simulink library "microgridLibrary"  (R2019b)
settings: Solver=VariableStepAuto  StartTime=0.0  StopTime=10.0  RelTol=1e-3
undefined symbols (not defined in the file or in its folder): Aa, BR, D1, Delta, DiscIntNeverNeededParam, Fn, gcbh, Ion, kv, Lithium, Ls, Pa, Pb, Pc, Rs, sps_rtmsupport, StationData, Ts, Ts_Control, Vn, Vnom
libraries: powerlib x80, simulink x29, powerlib_meascontrol x28, sps_avr x5, spsDieselMotorModel x3, electricdrivelib x2, re_lib x1
(part 4 of 6)

== system microgridLibrary/Solar Array (EMT Model)/Inverter Control ==
  On : Inport  PortDimensions=1
  Vabc_prim : Inport  Port=2  PortDimensions=3
  Iabc_prim : Inport  Port=3  PortDimensions=3
  V_PV : Inport  Port=4  PortDimensions=1
  I_PV : Inport  Port=5  PortDimensions=1
  Vdc_meas : Inport  Port=6  PortDimensions=1
  Current Regulator : Subsystem
  Iq_ref : Constant  Value=0
  MPPT Parameters : Subsystem
  "MPPT Controller using Perturbe & Observe technique " : MATLAB Function  TreatAsAtomicUnit=on
  Mux : Mux  Inputs=2
  Overmodulation : powerlib_meascontrol/Pulse & Signal Generators/Overmodulation  OverModType=Flat top
      settings: SourceProductName=Simscape Electrical  SourceProductBaseCode=PS
  PLL & Measurements : Subsystem
  Switch : Switch  Criteria=u2 ~= 0
  Uabc_ref Generation max (m) = 1 : Subsystem
  Unit Delay : UnitDelay  SampleTime=Ts_Control  HasFrameUpgradeWarning=on
  VDC Regulator : Subsystem
  Vnom_dc1 : Constant  Value=Vnom_dc
  Uref : Outport  VectorParamsAs1DForOutWhenUnconnected=off
  wires:
  PLL & Measurements/1(wt) -> Uabc_ref Generation max (m) = 1/1(wt)
  Current Regulator/1(VdVq_conv) -> Uabc_ref Generation max (m) = 1/2(VdVq_conv)
  Iq_ref/1 -> Mux/2
  Mux/1 -> Current Regulator/3(IdIq_ref)
  PLL & Measurements/3(IdIq_prim) -> Current Regulator/2(IdIq_meas)
  PLL & Measurements/2(VdVq_prim) -> Current Regulator/1(VdVq_meas)
  Vabc_prim/1 -> PLL & Measurements/1(Vabc_prim)
  Iabc_prim/1 -> PLL & Measurements/2(Iabc_prim)
  Overmodulation/1 -> Uref/1
  Vdc_meas/1 -> VDC Regulator/1(Vdc_meas)
  VDC Regulator/1(Id_ref) -> Mux/1
  V_PV/1 -> "MPPT Controller using Perturbe & Observe technique "/3(V)
  I_PV/1 -> "MPPT Controller using Perturbe & Observe technique "/4(I)
  MPPT Parameters/1(Param) -> "MPPT Controller using Perturbe & Observe technique "/1(Param)
  On/1 -> "MPPT Controller using Perturbe & Observe technique "/2(Enabled), Switch/2
  Unit Delay/1 -> Overmodulation/1
  "MPPT Controller using Perturbe & Observe technique "/1(D) -> Switch/1
  Switch/1 -> VDC Regulator/2(Vdc_ref)
  Vnom_dc1/1 -> Switch/3
  Uabc_ref Generation max (m) = 1/1(Uabc_ref) -> Unit Delay/1

== system microgridLibrary/Solar Array (EMT Model)/Measures ==
  Grid : Inport
  PV : Inport  Port=2
  Bus Creator : BusCreator  Inputs=2
  Bus Creator1 : BusCreator  Inputs=4
  Bus Selector2 : BusSelector  OutputSignals=Vabc,Iabc
  "Power (3ph, Instantaneous)" : powerlib_meascontrol/Measurements/Power (3ph, Instantaneous)
      settings: SourceProductName=Simscape Electrical
  m : Outport  VectorParamsAs1DForOutWhenUnconnected=off
  wires:
  Bus Selector2/1 -> "Power (3ph, Instantaneous)"/1, Bus Creator1/1  "<Vabc>"
  Bus Selector2/2 -> "Power (3ph, Instantaneous)"/2, Bus Creator1/2  "<Iabc>"
  "Power (3ph, Instantaneous)"/1 -> Bus Creator1/3  "P"
  Bus Creator/1 -> m/1
  PV/1 -> Bus Creator/2  "PV"
  Grid/1 -> Bus Selector2/1
  "Power (3ph, Instantaneous)"/2 -> Bus Creator1/4  "Q"
  Bus Creator1/1 -> Bus Creator/1  "Grid"

== system microgridLibrary/Variable Load/Dynamic Load Control ==
  P0 : Inport
  Fcn : Fcn  Expr=sqrt(1/u(1)-1)
  Mux : Mux  Inputs=2
  Product : Product
  Summer1 : Constant  Value=PF
  PQ : Outport  VectorParamsAs1DForOutWhenUnconnected=off
  wires:
  Summer1/1 -> Fcn/1
  Fcn/1 -> Product/2
  P0/1 -> Product/1, Mux/1
  Mux/1 -> PQ/1
  Product/1 -> Mux/2  "Qo"

== system microgridLibrary/Diesel Generator (Full Genset Controls)/Continuous/Automatic Generator Controls ==
  Mode : Inport
  PQwv_ref : Inport  Port=2
  GenM : Inport  Port=3
  Demux : Demux  Outputs=2
  "Direct wref, Vref" : Selector  InputPortWidth=4  IndexOptions=Index vector (dialog)  Indices=[3 4]  OutputSizes=1
  Multiport Switch : MultiPortSwitch  DataPortOrder=Zero-based contiguous  zeroidx=on
  PQ Control : Subsystem
  PV Control : Subsystem
  wref : Outport  VectorParamsAs1DForOutWhenUnconnected=off
  vref : Outport  Port=2  VectorParamsAs1DForOutWhenUnconnected=off
  wires:
  Mode/1 -> Multiport Switch/1
  PQwv_ref/1 -> PV Control/1(PQ_wv_ref), "Direct wref, Vref"/1, PQ Control/1(PQ_wv_ref)
  GenM/1 -> PV Control/2(GenM), PQ Control/2(GenM)
  "Direct wref, Vref"/1 -> Multiport Switch/2
  PQ Control/1("wref, Vref") -> Multiport Switch/3
  PV Control/1("wref, Vref") -> Multiport Switch/4
  Multiport Switch/1 -> Demux/1
  Demux/1 -> wref/1
  Demux/2 -> vref/1

== system microgridLibrary/Diesel Generator (Full Genset Controls)/Continuous/Generator Measures ==
  m : Inport
  Bus Selector : BusSelector  OutputSignals="dq0 components.Stator voltage  vq (pu),dq0 components.Stator voltage  vd (pu)"  OutputAsBus=on
  Bus Selector1 : BusSelector  OutputSignals="Mechanical.Rotor speed  wm  (pu),dq0 components.Field current  ifd (pu)"
  Fcn1 : Fcn  Expr=sqrt(u(1)^2 + u(2)^2)
  Ifd : Outport  VectorParamsAs1DForOutWhenUnconnected=off
  Vt : Outport  Port=2  VectorParamsAs1DForOutWhenUnconnected=off
  wm : Outport  Port=3  VectorParamsAs1DForOutWhenUnconnected=off
  wires:
  Fcn1/1 -> Vt/1
  Bus Selector1/2 -> Ifd/1  "<Field current  ifd (pu)>"
  Bus Selector/1 -> Fcn1/1
  m/1 -> Bus Selector/1, Bus Selector1/1
  Bus Selector1/1 -> wm/1  "<Rotor speed  wm  (pu)>"

== system microgridLibrary/Diesel Generator (Full Genset Controls)/Continuous/Selected Measurements ==
  m : Inport
  Bus Creator : BusCreator  Inputs=7
  Bus Selector : BusSelector  OutputSignals="Mechanical.Electrical power  Pe (pu),Mechanical.Rotor speed  wm  (pu),Output active power   Peo (pu),Output reactive power  Qeo (pu)"
  to W : Gain  Gain=Pn
  to W1 : Gain  Gain=Pn
  to W2 : Gain  Gain=Pn
  sm : Outport  VectorParamsAs1DForOutWhenUnconnected=off
  wires:
  m/1 -> Bus Selector/1
  Bus Selector/4 -> to W2/1, Bus Creator/5  "<Output reactive power  Qeo (pu)>"
  Bus Selector/1 -> Bus Creator/2, to W/1  "<Electrical power  Pe (pu)>"
  Bus Selector/3 -> to W1/1, Bus Creator/4  "<Output active power   Peo (pu)>"
  to W/1 -> Bus Creator/1  "Electrical Power (W)"
  Bus Creator/1 -> sm/1
  Bus Selector/2 -> Bus Creator/3  "<Rotor speed  wm  (pu)>"
  to W1/1 -> Bus Creator/6  "Active Power (W)"
  to W2/1 -> Bus Creator/7  "Reactive Power (W)"

== system microgridLibrary/Diesel Generator (Full Genset Controls)/Discrete/Automatic Generator Controls ==
  Mode : Inport
  PQwv_ref : Inport  Port=2  SampleTime=Ts
  GenM : Inport  Port=3
  Demux : Demux  Outputs=2
  "Direct wref, Vref" : Selector  InputPortWidth=4  IndexOptions=Index vector (dialog)  Indices=[3 4]  OutputSizes=1
  Multiport Switch : MultiPortSwitch  DataPortOrder=Zero-based contiguous  zeroidx=on
  PQ Control : Subsystem
  PV Control : Subsystem
  wref : Outport  VectorParamsAs1DForOutWhenUnconnected=off
  vref : Outport  Port=2  VectorParamsAs1DForOutWhenUnconnected=off
  wires:
  Mode/1 -> Multiport Switch/1
  PQwv_ref/1 -> PV Control/1(PQ_wv_ref), "Direct wref, Vref"/1, PQ Control/1(PQ_wv_ref)
  GenM/1 -> PV Control/2(GenM), PQ Control/2(GenM)
  "Direct wref, Vref"/1 -> Multiport Switch/2
  PQ Control/1("wref, Vref") -> Multiport Switch/3
  PV Control/1("wref, Vref") -> Multiport Switch/4
  Multiport Switch/1 -> Demux/1
  Demux/1 -> wref/1
  Demux/2 -> vref/1

== system microgridLibrary/Diesel Generator (Full Genset Controls)/Discrete/Diesel Engine Governor ==
  note: ACTUATOR
  wref (pu) : Inport  SampleTime=Ts
  w (pu) : Inport  Port=2  SampleTime=Ts
  CONTROL SYSTEM : Subsystem
      mask Display: fprintf('(Tr3s + 1)\n-------------------------\n(1+sTr1 + s^2 Tr1*Tr2)');
  ENGINE Td : Delay  DelayLength=ceil(Td/Ts)  InitialCondition=Pm0
  Gain K : Gain  Gain=K  SaturateOnIntegerOverflow=on  OutDataTypeStr=Inherit: Same as input  ParamDataTypeStr=Inherit: Same as input
  Integrator : DiscreteIntegrator  InitialCondition=Pm0  SampleTime=Ts  LimitOutput=on  UpperSaturationLimit=Tlim(2)  LowerSaturationLimit=Tlim(1)  ICPrevOutput=DiscIntNeverNeededParam  ICPrevScaledInput=DiscIntNeverNeededParam
  Product : Product  SaturateOnIntegerOverflow=on  InputSameDT=on  OutDataTypeStr=Inherit: Same as first input
  Sum : Sum  Inputs=+-  SaturateOnIntegerOverflow=on  InputSameDT=on  OutDataTypeStr=Inherit: Same as first input
  TF1 : Subsystem
      mask Display: fprintf('(1 + s Ta1)\n------------\n(1 + s Ta2)');
  TF2 : Subsystem
      mask Display: fprintf('1\n------------\n(1 + s Ta3)');
  Pmec (pu) : Outport  InitialOutput=0  VectorParamsAs1DForOutWhenUnconnected=off
  wires:
  Gain K/1 -> TF1/1(In1)
  Sum/1 -> CONTROL SYSTEM/1(In1)
  CONTROL SYSTEM/1(Out1) -> Gain K/1
  TF1/1(Out1) -> TF2/1(In1)
  w (pu)/1 -> Product/2, Sum/2
  ENGINE Td/1 -> Product/1
  wref (pu)/1 -> Sum/1
  Product/1 -> Pmec (pu)/1
  TF2/1(Out1) -> Integrator/1
  Integrator/1 -> ENGINE Td/1  "Torque"

== system microgridLibrary/Diesel Generator (Full Genset Controls)/Discrete/Generator Measures ==
  m : Inport
  Bus Selector : BusSelector  OutputSignals="dq0 components.Stator voltage  vq (pu),dq0 components.Stator voltage  vd (pu)"  OutputAsBus=on
  Bus Selector1 : BusSelector  OutputSignals="Mechanical.Rotor speed  wm  (pu),dq0 components.Field current  ifd (pu)"
  Fcn1 : Fcn  Expr=sqrt(u(1)^2 + u(2)^2)
  Ifd : Outport  VectorParamsAs1DForOutWhenUnconnected=off
  Vt : Outport  Port=2  VectorParamsAs1DForOutWhenUnconnected=off
  wm : Outport  Port=3  VectorParamsAs1DForOutWhenUnconnected=off
  wires:
  Bus Selector1/1 -> wm/1  "<Rotor speed  wm  (pu)>"
  m/1 -> Bus Selector1/1, Bus Selector/1
  Fcn1/1 -> Vt/1
  Bus Selector/1 -> Fcn1/1
  Bus Selector1/2 -> Ifd/1  "<Field current  ifd (pu)>"

== system microgridLibrary/Diesel Generator (Full Genset Controls)/Discrete/Selected Measurements ==
  m : Inport
  Bus Creator : BusCreator  Inputs=7
  Bus Selector : BusSelector  OutputSignals="Mechanical.Electrical power  Pe (pu),Mechanical.Rotor speed  wm  (pu),Output active power   Peo (pu),Output reactive power  Qeo (pu)"
  to W : Gain  Gain=Pn
  to W1 : Gain  Gain=Pn
  to W2 : Gain  Gain=Pn
  sm : Outport  VectorParamsAs1DForOutWhenUnconnected=off
  wires:
  to W2/1 -> Bus Creator/7  "Reactive Power (W)"
  to W1/1 -> Bus Creator/6  "Active Power (W)"
  Bus Selector/2 -> Bus Creator/3  "<Rotor speed  wm  (pu)>"
  Bus Creator/1 -> sm/1
  to W/1 -> Bus Creator/1  "Electrical Power (W)"
  Bus Selector/3 -> Bus Creator/4, to W1/1  "<Output active power   Peo (pu)>"
  Bus Selector/1 -> to W/1, Bus Creator/2  "<Electrical power  Pe (pu)>"
  Bus Selector/4 -> Bus Creator/5, to W2/1  "<Output reactive power  Qeo (pu)>"
  m/1 -> Bus Selector/1

== system microgridLibrary/Diesel Generator (Simple Controls)/Continuous/Generator Measures ==
  m : Inport
  Bus Selector : BusSelector  OutputSignals="dq0 components.Stator voltage  vq (pu),dq0 components.Stator voltage  vd (pu)"  OutputAsBus=on
  Bus Selector1 : BusSelector  OutputSignals="Mechanical.Rotor speed  wm  (pu),dq0 components.Field current  ifd (pu)"
  Fcn1 : Fcn  Expr=sqrt(u(1)^2 + u(2)^2)
  Ifd : Outport  VectorParamsAs1DForOutWhenUnconnected=off
  Vt : Outport  Port=2  VectorParamsAs1DForOutWhenUnconnected=off
  wm : Outport  Port=3  VectorParamsAs1DForOutWhenUnconnected=off
  wires:
  Bus Selector1/1 -> wm/1  "<Rotor speed  wm  (pu)>"
  m/1 -> Bus Selector1/1, Bus Selector/1
  Bus Selector/1 -> Fcn1/1
  Bus Selector1/2 -> Ifd/1  "<Field current  ifd (pu)>"
  Fcn1/1 -> Vt/1

== system microgridLibrary/Diesel Generator (Simple Controls)/Continuous/Selected Measurements ==
  m : Inport
  Bus Creator : BusCreator  Inputs=7
  Bus Selector : BusSelector  OutputSignals="Mechanical.Electrical power  Pe (pu),Mechanical.Rotor speed  wm  (pu),Output active power   Peo (pu),Output reactive power  Qeo (pu)"
  to W : Gain  Gain=Pn
  to W1 : Gain  Gain=Pn
  to W2 : Gain  Gain=Pn
  sm : Outport  VectorParamsAs1DForOutWhenUnconnected=off
  wires:
  to W2/1 -> Bus Creator/7  "Reactive Power (W)"
  to W1/1 -> Bus Creator/6  "Active Power (W)"
  Bus Selector/2 -> Bus Creator/3  "<Rotor speed  wm  (pu)>"
  Bus Creator/1 -> sm/1
  to W/1 -> Bus Creator/1  "Electrical Power (W)"
  Bus Selector/3 -> Bus Creator/4, to W1/1  "<Output active power   Peo (pu)>"
  Bus Selector/1 -> to W/1, Bus Creator/2  "<Electrical power  Pe (pu)>"
  Bus Selector/4 -> Bus Creator/5, to W2/1  "<Output reactive power  Qeo (pu)>"
  m/1 -> Bus Selector/1

== system microgridLibrary/Diesel Generator (Simple Controls)/Discrete/Diesel Engine Governor ==
  note: ACTUATOR
  wref (pu) : Inport  SampleTime=Ts
  w (pu) : Inport  Port=2  SampleTime=Ts
  CONTROL SYSTEM : Subsystem
      mask Display: fprintf('(Tr3s + 1)\n-------------------------\n(1+sTr1 + s^2 Tr1*Tr2)');
  ENGINE Td : Delay  DelayLength=ceil(Td/Ts)  InitialCondition=Pm0
  Gain K : Gain  Gain=K  SaturateOnIntegerOverflow=on  OutDataTypeStr=Inherit: Same as input  ParamDataTypeStr=Inherit: Same as input
  Integrator : DiscreteIntegrator  InitialCondition=Pm0  SampleTime=Ts  LimitOutput=on  UpperSaturationLimit=Tlim(2)  LowerSaturationLimit=Tlim(1)  ICPrevOutput=DiscIntNeverNeededParam  ICPrevScaledInput=DiscIntNeverNeededParam
  Product : Product  SaturateOnIntegerOverflow=on  InputSameDT=on  OutDataTypeStr=Inherit: Same as first input
  Sum : Sum  Inputs=+-  SaturateOnIntegerOverflow=on  InputSameDT=on  OutDataTypeStr=Inherit: Same as first input
  TF1 : Subsystem
      mask Display: fprintf('(1 + s Ta1)\n------------\n(1 + s Ta2)');
  TF2 : Subsystem
      mask Display: fprintf('1\n------------\n(1 + s Ta3)');
  Pmec (pu) : Outport  InitialOutput=0  VectorParamsAs1DForOutWhenUnconnected=off
  wires:
  Integrator/1 -> ENGINE Td/1  "Torque"
  TF2/1(Out1) -> Integrator/1
  Product/1 -> Pmec (pu)/1
  wref (pu)/1 -> Sum/1
  ENGINE Td/1 -> Product/1
  w (pu)/1 -> Sum/2, Product/2
  TF1/1(Out1) -> TF2/1(In1)
  CONTROL SYSTEM/1(Out1) -> Gain K/1
  Sum/1 -> CONTROL SYSTEM/1(In1)
  Gain K/1 -> TF1/1(In1)

== system microgridLibrary/Diesel Generator (Simple Controls)/Discrete/Generator Measures ==
  m : Inport
  Bus Selector : BusSelector  OutputSignals="dq0 components.Stator voltage  vq (pu),dq0 components.Stator voltage  vd (pu)"  OutputAsBus=on
  Bus Selector1 : BusSelector  OutputSignals="Mechanical.Rotor speed  wm  (pu),dq0 components.Field current  ifd (pu)"
  Fcn1 : Fcn  Expr=sqrt(u(1)^2 + u(2)^2)
  Ifd : Outport  VectorParamsAs1DForOutWhenUnconnected=off
  Vt : Outport  Port=2  VectorParamsAs1DForOutWhenUnconnected=off
  wm : Outport  Port=3  VectorParamsAs1DForOutWhenUnconnected=off
  wires:
  Bus Selector1/2 -> Ifd/1  "<Field current  ifd (pu)>"
  Bus Selector/1 -> Fcn1/1
  Fcn1/1 -> Vt/1
  m/1 -> Bus Selector/1, Bus Selector1/1
  Bus Selector1/1 -> wm/1  "<Rotor speed  wm  (pu)>"

== system microgridLibrary/Diesel Generator (Simple Controls)/Discrete/Selected Measurements ==
  m : Inport
  Bus Creator : BusCreator  Inputs=7
  Bus Selector : BusSelector  OutputSignals="Mechanical.Electrical power  Pe (pu),Mechanical.Rotor speed  wm  (pu),Output active power   Peo (pu),Output reactive power  Qeo (pu)"
  to W : Gain  Gain=Pn
  to W1 : Gain  Gain=Pn
  to W2 : Gain  Gain=Pn
  sm : Outport  VectorParamsAs1DForOutWhenUnconnected=off
  wires:
  m/1 -> Bus Selector/1
  Bus Selector/4 -> to W2/1, Bus Creator/5  "<Output reactive power  Qeo (pu)>"
  Bus Selector/1 -> Bus Creator/2, to W/1  "<Electrical power  Pe (pu)>"
  Bus Selector/3 -> to W1/1, Bus Creator/4  "<Output active power   Peo (pu)>"
  to W/1 -> Bus Creator/1  "Electrical Power (W)"
  Bus Creator/1 -> sm/1
  Bus Selector/2 -> Bus Creator/3  "<Rotor speed  wm  (pu)>"
  to W1/1 -> Bus Creator/6  "Active Power (W)"
  to W2/1 -> Bus Creator/7  "Reactive Power (W)"

== system microgridLibrary/Energy Storage (PQ Model)/Charge Limits/Overcharge Check ==
  SOC (%) : Inport
  Pin : Inport  Port=2
  Qin : Inport  Port=3
  Backlash : Backlash  BacklashWidth=1e-3  InitialOutput=Initial_kWh_pc  ZeroCross=off
  Compare To Constant : simulink/Logic and Bit Operations/Compare To Constant  relop=>  const=UpChrgLim  OutDataTypeStr=boolean
  Compare To Zero : simulink/Logic and Bit Operations/Compare To Zero  relop=<=  OutDataTypeStr=boolean
  Constant : Constant  Value=0
  Constant1 : Constant  Value=0
  Logical Operator : Logic  AllPortsSameDT=off  OutDataTypeStr=boolean
  Switch : Switch  Criteria=u2 ~= 0
  Switch1 : Switch  Criteria=u2 ~= 0
  Pout : Outport  VectorParamsAs1DForOutWhenUnconnected=off
  Qout : Outport  Port=2  VectorParamsAs1DForOutWhenUnconnected=off
  wires:
  Backlash/1 -> Compare To Constant/1
  Switch1/1 -> Qout/1
  Constant1/1 -> Switch1/1
  Qin/1 -> Switch1/3
  Compare To Zero/1 -> Logical Operator/2
  Switch/1 -> Pout/1
  Pin/1 -> Switch/3, Compare To Zero/1
  SOC (%)/1 -> Backlash/1
  Constant/1 -> Switch/1
  Logical Operator/1 -> Switch/2, Switch1/2
  Compare To Constant/1 -> Logical Operator/1

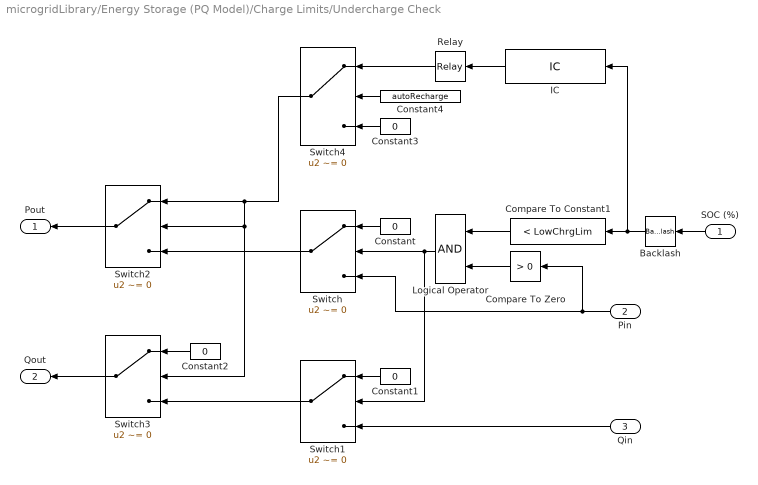
== system microgridLibrary/Energy Storage (PQ Model)/Charge Limits/Undercharge Check ==
  SOC (%) : Inport
  Pin : Inport  Port=2
  Qin : Inport  Port=3
  Backlash : Backlash  BacklashWidth=1e-3  InitialOutput=Initial_kWh_pc  ZeroCross=off
  Compare To Constant1 : simulink/Logic and Bit Operations/Compare To Constant  relop=<  const=LowChrgLim  OutDataTypeStr=boolean
  Compare To Zero : simulink/Logic and Bit Operations/Compare To Zero  relop=>  OutDataTypeStr=boolean
  Constant{,1..3} (4 alike) : Constant  Value=0
  Constant4 : Constant  Value=autoRecharge
  IC : InitialCondition  Value=RechargeSOC
  Logical Operator : Logic  AllPortsSameDT=off  OutDataTypeStr=boolean
  Relay : Relay  OnSwitchValue=RechargeSOC  OffSwitchValue=LowChrgLim  OnOutputValue=0  OffOutputValue=-Precharge/100*Pnom
  Switch{,1..4} (5 alike) : Switch  Criteria=u2 ~= 0
  Pout : Outport  VectorParamsAs1DForOutWhenUnconnected=off
  Qout : Outport  Port=2  VectorParamsAs1DForOutWhenUnconnected=off
  wires:
  Constant4/1 -> Switch4/2
  Constant3/1 -> Switch4/3
  Relay/1 -> Switch4/1
  Constant2/1 -> Switch3/1
  Switch1/1 -> Switch3/3
  Switch3/1 -> Qout/1
  Switch2/1 -> Pout/1
  Switch/1 -> Switch2/3
  IC/1 -> Relay/1
  Switch4/1 -> Switch3/2, Switch2/2, Switch2/1
  Backlash/1 -> Compare To Constant1/1, IC/1
  Qin/1 -> Switch1/3
  Constant1/1 -> Switch1/1
  Compare To Constant1/1 -> Logical Operator/1
  Logical Operator/1 -> Switch1/2, Switch/2
  Constant/1 -> Switch/1
  SOC (%)/1 -> Backlash/1
  Pin/1 -> Compare To Zero/1, Switch/3
  Compare To Zero/1 -> Logical Operator/2

== system microgridLibrary/Energy Storage (PQ Model)/Power Measures/EMT ==
  "Power (3ph, Instantaneous)" : powerlib_meascontrol/Measurements/Power (3ph, Instantaneous)
      settings: SourceProductName=Simscape Electrical
  Three-Phase V-I Measurement : powerlib/Measurements/Three-Phase V-I Measurement  VoltageMeasurement=phase-to-ground  SetLabelV=off  LabelV=Vabc  Vpu=off  VpuLL=off  CurrentMeasurement=yes  SetLabelI=off  LabelI=Iabc  Ipu=off  Pbase=100e6  Vbase=500e3  OutputType=Complex  PhasorSimulation=on  PSBequivalent=0
      settings: SourceProductName=Simscape Electrical
  A : PMIOPort  Side=Left
  a : PMIOPort  Port=2  Side=Right
  B : PMIOPort  Port=3  Side=Left
  b : PMIOPort  Port=4  Side=Right
  C : PMIOPort  Port=5  Side=Left
  c : PMIOPort  Port=6  Side=Right
  P : Outport  VectorParamsAs1DForOutWhenUnconnected=off
  Q : Outport  Port=2  VectorParamsAs1DForOutWhenUnconnected=off
  wires:
  Three-Phase V-I Measurement/2 -> "Power (3ph, Instantaneous)"/2
  Three-Phase V-I Measurement/1 -> "Power (3ph, Instantaneous)"/1
  "Power (3ph, Instantaneous)"/1 -> P/1
  "Power (3ph, Instantaneous)"/2 -> Q/1
  connections:
  Three-Phase V-I Measurement/RConn1 -- a/RConn1
  b/RConn1 -- Three-Phase V-I Measurement/RConn2
  A/RConn1 -- Three-Phase V-I Measurement/LConn1
  Three-Phase V-I Measurement/LConn2 -- B/RConn1
  c/RConn1 -- Three-Phase V-I Measurement/RConn3
  C/RConn1 -- Three-Phase V-I Measurement/LConn3

== system microgridLibrary/Energy Storage (PQ Model)/Power Measures/Phasor ==
  "Power (3ph, Phasor)" : powerlib_meascontrol/Measurements/Power (3ph, Phasor)
      settings: SourceProductName=Simscape Electrical  SourceProductBaseCode=PS
  Three-Phase V-I Measurement : powerlib/Measurements/Three-Phase V-I Measurement  VoltageMeasurement=phase-to-ground  SetLabelV=off  LabelV=Vabc  Vpu=off  VpuLL=off  CurrentMeasurement=yes  SetLabelI=off  LabelI=Iabc  Ipu=off  Pbase=100e6  Vbase=500e3  OutputType=Complex  PhasorSimulation=on  PSBequivalent=0
      settings: SourceProductName=Simscape Electrical
  A : PMIOPort  Side=Left
  a : PMIOPort  Port=2  Side=Right
  B : PMIOPort  Port=3  Side=Left
  b : PMIOPort  Port=4  Side=Right
  C : PMIOPort  Port=5  Side=Left
  c : PMIOPort  Port=6  Side=Right
  P : Outport  VectorParamsAs1DForOutWhenUnconnected=off
  Q : Outport  Port=2  VectorParamsAs1DForOutWhenUnconnected=off
  wires:
  "Power (3ph, Phasor)"/2 -> Q/1
  "Power (3ph, Phasor)"/1 -> P/1
  Three-Phase V-I Measurement/1 -> "Power (3ph, Phasor)"/1
  Three-Phase V-I Measurement/2 -> "Power (3ph, Phasor)"/2
  connections:
  C/RConn1 -- Three-Phase V-I Measurement/LConn3
  c/RConn1 -- Three-Phase V-I Measurement/RConn3
  Three-Phase V-I Measurement/LConn2 -- B/RConn1
  A/RConn1 -- Three-Phase V-I Measurement/LConn1
  b/RConn1 -- Three-Phase V-I Measurement/RConn2
  Three-Phase V-I Measurement/RConn1 -- a/RConn1

== system microgridLibrary/Fault /Fault A/Model ==
  "gate " : Inport
  Uswitch : Inport  Port=2
  C4 : Constant  Value=BR.com
  Data Type Conversion : DataTypeConversion  OutDataTypeStr=double  SaturateOnIntegerOverflow=on  RndMeth=Zero
  Switch3 : Switch  Threshold=0.5  ZeroCross=off  InputSameDT=on
  This signal is not used : Terminator
  Timer : Subsystem  DialogController=POWERSYS.PowerSysDialog  mask(Timer){t=BR.SwitchingTimes, e=BR.switchings}
      mask prompts: t "Time (s):"; e "Amplitude:"
      mask help:
      | Generates a signal changing at specified times.
      |
      | If a signal value is not specified at time zero, the output is kept at 0 until the first specified transition time.
      mask init:
      | tt=t;
      | sv=e;
      | if isempty(tt) | isempty(sv)
      | 	% probably during the load process when under a masked block.
      | 	tt=0;
      | 	sv=1;
      | end
      | %
      | if length(sv) ~= length(tt),
      |    Erreur.message = 'The vectors specifying the time and amplitude pairs must have the same length.';
      |    Erreur.identifier = 'SimscapePowerSystemsST:TimerBlock:ParameterError';
      |    powericon('psberror',Erreur.message,Erreur.identifier,'NoUiwait');
      | end
      | if tt(1)~=0,
      |    tt=[0 tt];
      |    sv=[~sv(1) sv];
      | end
      | n=length(tt);
      | vec_dt=[tt,0]-[0,tt] ;
      | vec_dt=vec_dt(2:n);
      | if any(vec_dt<=0)
      |    Erreur.message = 'All transition times must be in increasing order.';
      |    Erreur.identifier = 'SimscapePowerSystemsST:TimerBlock:ParameterError';
      |    powericon('psberror',Erreur.message,Erreur.identifier,'NoUiwait');
      | end
      | tv=[-1,tt(1),reshape(repmat(reshape(tt(2:end),1,length(tt)-1),2,1),1,2*length(tt)-2),tt(end)+1];
      | %sv=(sv(:)'~=0);
      | opv=[sv(1),reshape(repmat(sv(1:end-1),2,1),1,2*length(sv)-2),sv(end),sv(end)];
      | 
      | power_initmask();
      mask Help: helpview(psbhelp)
      mask Display: plot( tv(2:end-1), opv(2:end-1) )
  gate : Outport  VectorParamsAs1DForOutWhenUnconnected=off
  wires:
  Uswitch/1 -> This signal is not used/1
  C4/1 -> Switch3/2
  Timer/1(Out) -> Switch3/3
  Data Type Conversion/1 -> Switch3/1
  Switch3/1 -> gate/1
  "gate "/1 -> Data Type Conversion/1

== system microgridLibrary/Fault /Fault B/Model ==
  "gate " : Inport
  Uswitch : Inport  Port=2
  C4 : Constant  Value=BR.com
  Data Type Conversion : DataTypeConversion  OutDataTypeStr=double  SaturateOnIntegerOverflow=on  RndMeth=Zero
  Switch3 : Switch  Threshold=0.5  ZeroCross=off  InputSameDT=on
  This signal is not used : Terminator
  Timer : Subsystem  DialogController=POWERSYS.PowerSysDialog  mask(Timer){t=BR.SwitchingTimes, e=BR.switchings}
      mask prompts: t "Time (s):"; e "Amplitude:"
      mask help:
      | Generates a signal changing at specified times.
      |
      | If a signal value is not specified at time zero, the output is kept at 0 until the first specified transition time.
      mask init: same as microgridLibrary/Fault /Fault A/Model/Timer
      mask Help: helpview(psbhelp)
      mask Display: plot( tv(2:end-1), opv(2:end-1) )
  gate : Outport  VectorParamsAs1DForOutWhenUnconnected=off
  wires:
  Uswitch/1 -> This signal is not used/1
  C4/1 -> Switch3/2
  Timer/1(Out) -> Switch3/3
  Data Type Conversion/1 -> Switch3/1
  Switch3/1 -> gate/1
  "gate "/1 -> Data Type Conversion/1

== system microgridLibrary/Fault /Fault C/Model ==
  "gate " : Inport
  Uswitch : Inport  Port=2
  C4 : Constant  Value=BR.com
  Data Type Conversion : DataTypeConversion  OutDataTypeStr=double  SaturateOnIntegerOverflow=on  RndMeth=Zero
  Switch3 : Switch  Threshold=0.5  ZeroCross=off  InputSameDT=on
  This signal is not used : Terminator
  Timer : Subsystem  DialogController=POWERSYS.PowerSysDialog  mask(Timer){t=BR.SwitchingTimes, e=BR.switchings}
      mask prompts: t "Time (s):"; e "Amplitude:"
      mask help:
      | Generates a signal changing at specified times.
      |
      | If a signal value is not specified at time zero, the output is kept at 0 until the first specified transition time.
      mask init: same as microgridLibrary/Fault /Fault A/Model/Timer
      mask Help: helpview(psbhelp)
      mask Display: plot( tv(2:end-1), opv(2:end-1) )
  gate : Outport  VectorParamsAs1DForOutWhenUnconnected=off
  wires:
  Uswitch/1 -> This signal is not used/1
  C4/1 -> Switch3/2
  Timer/1(Out) -> Switch3/3
  Data Type Conversion/1 -> Switch3/1
  Switch3/1 -> gate/1
  "gate "/1 -> Data Type Conversion/1

== system microgridLibrary/Grid Source Phasor Load Flow/Model/Initial Voltage ==
  Constant3 : Constant  Value=0
  Integrator : Integrator  InitialCondition=0.95
  Aa : Outport
  wires:
  Constant3/1 -> Integrator/1
  Integrator/1 -> Aa/1

== system microgridLibrary/Grid-Connected Battery (EMT with Simple Controls)/Battery Controller/Compute PQ ==
  m : Inport
  Bus Selector : BusSelector  OutputSignals=Vabc,Iabc
  Mux : Mux  Inputs=2
  "Power (3ph, Instantaneous)" : powerlib_meascontrol/Measurements/Power (3ph, Instantaneous)
      settings: SourceProductName=Simscape Electrical
  to PU : Gain  Gain=1/Pnom
  "to PU " : Gain  Gain=1/Pnom
  PQm : Outport  VectorParamsAs1DForOutWhenUnconnected=off
  wires:
  Bus Selector/1 -> "Power (3ph, Instantaneous)"/1  "<Vabc>"
  "Power (3ph, Instantaneous)"/2 -> "to PU "/1
  Bus Selector/2 -> "Power (3ph, Instantaneous)"/2  "<Iabc>"
  "Power (3ph, Instantaneous)"/1 -> to PU/1
  m/1 -> Bus Selector/1
  to PU/1 -> Mux/1
  "to PU "/1 -> Mux/2
  Mux/1 -> PQm/1

== system microgridLibrary/Grid-Connected Battery (EMT with Simple Controls)/Battery Controller/P,Q Control  ==
  PQref : Inport
  m : Inport  Port=2
  Active Controller : simulink/Continuous/PID Controller  Controller=PI  Form=Parallel  TimeDomain=Discrete-time  SampleTime=Ts_Control  IntegratorMethod=Forward Euler  FilterMethod=Forward Euler  ControllerParametersSource=internal  P=1  I=10  D=0  UseFilter=on  N=100  TunerSelectOption=Transfer Function Based (PID Tuner App)  InitialConditionSource=internal  InitialConditionForIntegrator=0  InitialConditionForFilter=0  DifferentiatorICPrevScaledInput=0  ExternalReset=none  TrackingMode=off  Kt=1  LimitOutput=on  UpperSaturationLimit=1.5  LowerSaturationLimit=-1.5  LinearizeAsGain=off  AntiWindupMode=clamping  Kb=1  POutMin=[]  POutMax=[]  IOutMin=[]  IOutMax=[]  DOutMin=[]  DOutMax=[]  NOutMin=[]  NOutMax=[]  SumOutMin=[]  SumOutMax=[]  SaturationOutMin=[]  SaturationOutMax=[]  PParamMin=[]  PParamMax=[]  IParamMin=[]  IParamMax=[]  DParamMin=[]  DParamMax=[]  NParamMin=[]  NParamMax=[]  KbParamMin=[]  KbParamMax=[]  KtParamMin=[]  KtParamMax=[]  KbOutMin=[]  KbOutMax=[]  KtOutMin=[]  KtOutMax=[]  IntegratorOutMin=[]  IntegratorOutMax=[]  FilterOutMin=[]  FilterOutMax=[]  SumI1OutMin=[]  SumI1OutMax=[]  SumI2OutMin=[]  SumI2OutMax=[]  SumI3OutMin=[]  SumI3OutMax=[]  SumI4OutMin=[]  SumI4OutMax=[]  SumDOutMin=[]  SumDOutMax=[]  DifferentiatorOutMin=[]  DifferentiatorOutMax=[]  FilterDiffOutCoefMin=[]  FilterDiffOutCoefMax=[]  ReciprocalOutMin=[]  ReciprocalOutMax=[]  SumDenOutMin=[]  SumDenOutMax=[]  SumNumOutMin=[]  SumNumOutMax=[]  DivideOutMin=[]  DivideOutMax=[]  IntegratorContinuousStateAttributes=''  IntegratorStateMustResolveToSignalObject=off  IntegratorRTWStateStorageClass=Auto  FilterContinuousStateAttributes=''  FilterStateMustResolveToSignalObject=off  FilterRTWStateStorageClass=Auto  ParallelPVariant=InternalParameters  IdealPVariant=Disabled  IVariant=InternalParameters  DVariant=Disabled  IntegratorVariant=Discrete  SatVariant=Enabled  AWVariant=DiscClampingParallel  PCopyVariant=Disabled  TRVariant=Disabled  FdbkBlocksVariant=Forward  IdealPFdbkVariant=Disabled  SatFdbkVariant=Disabled  DerivativeFilterVariant=Disabled  NVariant=Disabled  NCopyVariant=Disabled_SignalSpec  FilterICVariant=Disabled  IntegratorICVariant=InternalICs  ExternalResetVariant=Disabled  TRSumVariant=Passthrough  SumFdbkVariant=Disabled  SumVariant=Sum_PI
  Demux : Demux  Outputs=2
  Demux1 : Demux  Outputs=2
  Mux : Mux  Inputs=2
  Reactive Controller : simulink/Continuous/PID Controller  Controller=PI  Form=Parallel  TimeDomain=Discrete-time  SampleTime=Ts_Control  IntegratorMethod=Forward Euler  FilterMethod=Forward Euler  ControllerParametersSource=internal  P=1  I=10  D=0  UseFilter=on  N=100  TunerSelectOption=Transfer Function Based (PID Tuner App)  InitialConditionSource=internal  InitialConditionForIntegrator=0  InitialConditionForFilter=0  DifferentiatorICPrevScaledInput=0  ExternalReset=none  TrackingMode=off  Kt=1  LimitOutput=on  UpperSaturationLimit=1.5  LowerSaturationLimit=-1.5  LinearizeAsGain=off  AntiWindupMode=clamping  Kb=1  POutMin=[]  POutMax=[]  IOutMin=[]  IOutMax=[]  DOutMin=[]  DOutMax=[]  NOutMin=[]  NOutMax=[]  SumOutMin=[]  SumOutMax=[]  SaturationOutMin=[]  SaturationOutMax=[]  PParamMin=[]  PParamMax=[]  IParamMin=[]  IParamMax=[]  DParamMin=[]  DParamMax=[]  NParamMin=[]  NParamMax=[]  KbParamMin=[]  KbParamMax=[]  KtParamMin=[]  KtParamMax=[]  KbOutMin=[]  KbOutMax=[]  KtOutMin=[]  KtOutMax=[]  IntegratorOutMin=[]  IntegratorOutMax=[]  FilterOutMin=[]  FilterOutMax=[]  SumI1OutMin=[]  SumI1OutMax=[]  SumI2OutMin=[]  SumI2OutMax=[]  SumI3OutMin=[]  SumI3OutMax=[]  SumI4OutMin=[]  SumI4OutMax=[]  SumDOutMin=[]  SumDOutMax=[]  DifferentiatorOutMin=[]  DifferentiatorOutMax=[]  FilterDiffOutCoefMin=[]  FilterDiffOutCoefMax=[]  ReciprocalOutMin=[]  ReciprocalOutMax=[]  SumDenOutMin=[]  SumDenOutMax=[]  SumNumOutMin=[]  SumNumOutMax=[]  DivideOutMin=[]  DivideOutMax=[]  IntegratorContinuousStateAttributes=''  IntegratorStateMustResolveToSignalObject=off  IntegratorRTWStateStorageClass=Auto  FilterContinuousStateAttributes=''  FilterStateMustResolveToSignalObject=off  FilterRTWStateStorageClass=Auto  ParallelPVariant=InternalParameters  IdealPVariant=Disabled  IVariant=InternalParameters  DVariant=Disabled  IntegratorVariant=Discrete  SatVariant=Enabled  AWVariant=DiscClampingParallel  PCopyVariant=Disabled  TRVariant=Disabled  FdbkBlocksVariant=Forward  IdealPFdbkVariant=Disabled  SatFdbkVariant=Disabled  DerivativeFilterVariant=Disabled  NVariant=Disabled  NCopyVariant=Disabled_SignalSpec  FilterICVariant=Disabled  IntegratorICVariant=InternalICs  ExternalResetVariant=Disabled  TRSumVariant=Passthrough  SumFdbkVariant=Disabled  SumVariant=Sum_PI
  Sum : Sum  Inputs=|+-
  Sum1 : Sum  Inputs=|-+
  Idq_ref : Outport  VectorParamsAs1DForOutWhenUnconnected=off
  wires:
  Sum1/1 -> Reactive Controller/1
  Sum/1 -> Active Controller/1
  Mux/1 -> Idq_ref/1
  Active Controller/1 -> Mux/1
  Reactive Controller/1 -> Mux/2
  Demux/2 -> Sum1/1  "Qref"
  Demux/1 -> Sum/1  "Pref"
  PQref/1 -> Demux/1
  m/1 -> Demux1/1
  Demux1/1 -> Sum/2
  Demux1/2 -> Sum1/2

== system microgridLibrary/Grid-Connected Battery (EMT with Simple Controls)/Inverter Control/Current Control ==
  wt : Inport
  VdVq_meas : Inport  Port=2  PortDimensions=2
  IdIq_meas : Inport  Port=3  PortDimensions=2
  IdIq_ref : Inport  Port=4  PortDimensions=2
  Current Regulator : Subsystem
  Uabc_ref Generation max (m) = 1 : Subsystem
  Uabc : Outport  VectorParamsAs1DForOutWhenUnconnected=off
  wires:
  Uabc_ref Generation max (m) = 1/1(Uabc_ref) -> Uabc/1
  IdIq_ref/1 -> Current Regulator/3(IdIq_ref)
  IdIq_meas/1 -> Current Regulator/2(IdIq_meas)
  VdVq_meas/1 -> Current Regulator/1(VdVq_meas)
  Current Regulator/1(VdVq_conv) -> Uabc_ref Generation max (m) = 1/2(VdVq_conv)
  wt/1 -> Uabc_ref Generation max (m) = 1/1(wt)

== system microgridLibrary/Grid-Connected Battery (EMT with Simple Controls)/Inverter Control/PLL & Measurements ==
  note: PLL & Measurements
      | ===================
  Vabc_prim : Inport
  Iabc_prim : Inport  Port=2
  PLL (3ph) : powerlib_meascontrol/PLL/PLL (3ph)  Fmin=45  Par_Init="[-0.57  Fnom]"  ParK=[180, 3200, 1]  TcD=Ts_Control  MaxRateChangeFreq=12  FilterCutOffFreq=25  Ts=Ts_Control  AGC=on
      settings: SourceProductName=Simscape Electrical
  Selector1 : Selector  InputPortWidth=3  IndexOptions=Index vector (dialog)  Indices=[1 2]  OutputSizes=1
  Selector2 : Selector  InputPortWidth=3  IndexOptions=Index vector (dialog)  Indices=[1 2]  OutputSizes=1
  Terminator : Terminator
  V->pu : Gain  Gain=1/(Vnom_prim*sqrt(2)/sqrt(3))  SaturateOnIntegerOverflow=on  OutDataTypeStr=Inherit: Same as input  ParamDataTypeStr=Inherit: Same as input
  V->pu1 : Gain  Gain=Vnom_prim*sqrt(3)/Pnom/sqrt(2)  SaturateOnIntegerOverflow=on  OutDataTypeStr=Inherit: Same as input  ParamDataTypeStr=Inherit: Same as input
  abc to dq0 : powerlib_meascontrol/Transformations/abc to dq0  Alignment=90 degrees behind phase A axis
      settings: SourceProductName=Simscape Electrical
  abc to dq1 : powerlib_meascontrol/Transformations/abc to dq0  Alignment=90 degrees behind phase A axis
      settings: SourceProductName=Simscape Electrical
  wt : Outport  VectorParamsAs1DForOutWhenUnconnected=off
  VdVq_prim : Outport  Port=2  VectorParamsAs1DForOutWhenUnconnected=off
  IdIq_prim : Outport  Port=3  VectorParamsAs1DForOutWhenUnconnected=off
  wires:
  V->pu1/1 -> abc to dq1/1
  V->pu/1 -> PLL (3ph)/1, abc to dq0/1
  abc to dq1/1 -> Selector1/1
  Vabc_prim/1 -> V->pu/1
  Iabc_prim/1 -> V->pu1/1
  abc to dq0/1 -> Selector2/1
  Selector2/1 -> VdVq_prim/1
  Selector1/1 -> IdIq_prim/1
  PLL (3ph)/2 -> wt/1, abc to dq1/2, abc to dq0/2
  PLL (3ph)/1 -> Terminator/1

== system microgridLibrary/Grid-Connected Battery (Multi-mode EMT Model)/Battery Controller/Compute PQ ==
  m : Inport
  Bus Selector : BusSelector  OutputSignals=Vabc,Iabc
  Mux : Mux  Inputs=2
  "Power (3ph, Instantaneous)" : powerlib_meascontrol/Measurements/Power (3ph, Instantaneous)
      settings: SourceProductName=Simscape Electrical
  to PU : Gain  Gain=1/Pnom
  "to PU " : Gain  Gain=1/Pnom
  PQm : Outport  VectorParamsAs1DForOutWhenUnconnected=off
  wires:
  Mux/1 -> PQm/1
  "to PU "/1 -> Mux/2
  to PU/1 -> Mux/1
  m/1 -> Bus Selector/1
  "Power (3ph, Instantaneous)"/1 -> to PU/1
  Bus Selector/2 -> "Power (3ph, Instantaneous)"/2  "<Iabc>"
  "Power (3ph, Instantaneous)"/2 -> "to PU "/1
  Bus Selector/1 -> "Power (3ph, Instantaneous)"/1  "<Vabc>"

== system microgridLibrary/Grid-Connected Battery (Multi-mode EMT Model)/Battery Controller/Disable Current Control ==
  Action Port : ActionPort  InitializeStates=reset
  Id_ref : Constant  Value=0
  Iq_ref : Constant  Value=0
  Mux : Mux  Inputs=2
  Idq_ref : Outport  VectorParamsAs1DForOutWhenUnconnected=off
  wires:
  Id_ref/1 -> Mux/1
  Iq_ref/1 -> Mux/2
  Mux/1 -> Idq_ref/1

== system microgridLibrary/Grid-Connected Battery (Multi-mode EMT Model)/Battery Controller/Frequency Control  ==
  m_freq : Inport
  Action Port : ActionPort  InitializeStates=reset
  Discrete PID Controller : simulink/Continuous/PID Controller  Controller=PI  Form=Parallel  TimeDomain=Discrete-time  SampleTime=Ts_Control  IntegratorMethod=Forward Euler  FilterMethod=Forward Euler  ControllerParametersSource=internal  P=0.1  I=0.01  D=0  UseFilter=on  N=100  TunerSelectOption=Transfer Function Based (PID Tuner App)  InitialConditionSource=internal  InitialConditionForIntegrator=0  InitialConditionForFilter=0  DifferentiatorICPrevScaledInput=0  ExternalReset=none  TrackingMode=off  Kt=1  LimitOutput=on  UpperSaturationLimit=1.5  LowerSaturationLimit=-1.5  LinearizeAsGain=off  AntiWindupMode=clamping  Kb=1  POutMin=[]  POutMax=[]  IOutMin=[]  IOutMax=[]  DOutMin=[]  DOutMax=[]  NOutMin=[]  NOutMax=[]  SumOutMin=[]  SumOutMax=[]  SaturationOutMin=[]  SaturationOutMax=[]  PParamMin=[]  PParamMax=[]  IParamMin=[]  IParamMax=[]  DParamMin=[]  DParamMax=[]  NParamMin=[]  NParamMax=[]  KbParamMin=[]  KbParamMax=[]  KtParamMin=[]  KtParamMax=[]  KbOutMin=[]  KbOutMax=[]  KtOutMin=[]  KtOutMax=[]  IntegratorOutMin=[]  IntegratorOutMax=[]  FilterOutMin=[]  FilterOutMax=[]  SumI1OutMin=[]  SumI1OutMax=[]  SumI2OutMin=[]  SumI2OutMax=[]  SumI3OutMin=[]  SumI3OutMax=[]  SumI4OutMin=[]  SumI4OutMax=[]  SumDOutMin=[]  SumDOutMax=[]  DifferentiatorOutMin=[]  DifferentiatorOutMax=[]  FilterDiffOutCoefMin=[]  FilterDiffOutCoefMax=[]  ReciprocalOutMin=[]  ReciprocalOutMax=[]  SumDenOutMin=[]  SumDenOutMax=[]  SumNumOutMin=[]  SumNumOutMax=[]  DivideOutMin=[]  DivideOutMax=[]  IntegratorContinuousStateAttributes=''  IntegratorStateMustResolveToSignalObject=off  IntegratorRTWStateStorageClass=Auto  FilterContinuousStateAttributes=''  FilterStateMustResolveToSignalObject=off  FilterRTWStateStorageClass=Auto  ParallelPVariant=InternalParameters  IdealPVariant=Disabled  IVariant=InternalParameters  DVariant=Disabled  IntegratorVariant=Discrete  SatVariant=Enabled  AWVariant=DiscClampingParallel  PCopyVariant=Disabled  TRVariant=Disabled  FdbkBlocksVariant=Forward  IdealPFdbkVariant=Disabled  SatFdbkVariant=Disabled  DerivativeFilterVariant=Disabled  NVariant=Disabled  NCopyVariant=Disabled_SignalSpec  FilterICVariant=Disabled  IntegratorICVariant=InternalICs  ExternalResetVariant=Disabled  TRSumVariant=Passthrough  SumFdbkVariant=Disabled  SumVariant=Sum_PI
  Frequency : Constant
  Iq_ref : Constant  Value=0
  Mux : Mux  Inputs=2
  Sum : Sum  Inputs=|+-
  Idq_ref : Outport  VectorParamsAs1DForOutWhenUnconnected=off
  wires:
  Mux/1 -> Idq_ref/1
  Iq_ref/1 -> Mux/2
  m_freq/1 -> Sum/2
  Frequency/1 -> Sum/1
  Sum/1 -> Discrete PID Controller/1
  Discrete PID Controller/1 -> Mux/1

== system microgridLibrary/Grid-Connected Battery (Multi-mode EMT Model)/Battery Controller/P,Q Control  ==
  PQref : Inport
  m : Inport  Port=2
  Action Port : ActionPort  InitializeStates=reset
  Active Controller : simulink/Continuous/PID Controller  Controller=PI  Form=Parallel  TimeDomain=Discrete-time  SampleTime=Ts_Control  IntegratorMethod=Forward Euler  FilterMethod=Forward Euler  ControllerParametersSource=internal  P=1  I=10  D=0  UseFilter=on  N=100  TunerSelectOption=Transfer Function Based (PID Tuner App)  InitialConditionSource=internal  InitialConditionForIntegrator=0  InitialConditionForFilter=0  DifferentiatorICPrevScaledInput=0  ExternalReset=none  TrackingMode=off  Kt=1  LimitOutput=on  UpperSaturationLimit=1.5  LowerSaturationLimit=-1.5  LinearizeAsGain=off  AntiWindupMode=clamping  Kb=1  POutMin=[]  POutMax=[]  IOutMin=[]  IOutMax=[]  DOutMin=[]  DOutMax=[]  NOutMin=[]  NOutMax=[]  SumOutMin=[]  SumOutMax=[]  SaturationOutMin=[]  SaturationOutMax=[]  PParamMin=[]  PParamMax=[]  IParamMin=[]  IParamMax=[]  DParamMin=[]  DParamMax=[]  NParamMin=[]  NParamMax=[]  KbParamMin=[]  KbParamMax=[]  KtParamMin=[]  KtParamMax=[]  KbOutMin=[]  KbOutMax=[]  KtOutMin=[]  KtOutMax=[]  IntegratorOutMin=[]  IntegratorOutMax=[]  FilterOutMin=[]  FilterOutMax=[]  SumI1OutMin=[]  SumI1OutMax=[]  SumI2OutMin=[]  SumI2OutMax=[]  SumI3OutMin=[]  SumI3OutMax=[]  SumI4OutMin=[]  SumI4OutMax=[]  SumDOutMin=[]  SumDOutMax=[]  DifferentiatorOutMin=[]  DifferentiatorOutMax=[]  FilterDiffOutCoefMin=[]  FilterDiffOutCoefMax=[]  ReciprocalOutMin=[]  ReciprocalOutMax=[]  SumDenOutMin=[]  SumDenOutMax=[]  SumNumOutMin=[]  SumNumOutMax=[]  DivideOutMin=[]  DivideOutMax=[]  IntegratorContinuousStateAttributes=''  IntegratorStateMustResolveToSignalObject=off  IntegratorRTWStateStorageClass=Auto  FilterContinuousStateAttributes=''  FilterStateMustResolveToSignalObject=off  FilterRTWStateStorageClass=Auto  ParallelPVariant=InternalParameters  IdealPVariant=Disabled  IVariant=InternalParameters  DVariant=Disabled  IntegratorVariant=Discrete  SatVariant=Enabled  AWVariant=DiscClampingParallel  PCopyVariant=Disabled  TRVariant=Disabled  FdbkBlocksVariant=Forward  IdealPFdbkVariant=Disabled  SatFdbkVariant=Disabled  DerivativeFilterVariant=Disabled  NVariant=Disabled  NCopyVariant=Disabled_SignalSpec  FilterICVariant=Disabled  IntegratorICVariant=InternalICs  ExternalResetVariant=Disabled  TRSumVariant=Passthrough  SumFdbkVariant=Disabled  SumVariant=Sum_PI
  Demux : Demux  Outputs=2
  Demux1 : Demux  Outputs=2
  Mux : Mux  Inputs=2
  Reactive Controller : simulink/Continuous/PID Controller  Controller=PI  Form=Parallel  TimeDomain=Discrete-time  SampleTime=Ts_Control  IntegratorMethod=Forward Euler  FilterMethod=Forward Euler  ControllerParametersSource=internal  P=1  I=10  D=0  UseFilter=on  N=100  TunerSelectOption=Transfer Function Based (PID Tuner App)  InitialConditionSource=internal  InitialConditionForIntegrator=0  InitialConditionForFilter=0  DifferentiatorICPrevScaledInput=0  ExternalReset=none  TrackingMode=off  Kt=1  LimitOutput=on  UpperSaturationLimit=1.5  LowerSaturationLimit=-1.5  LinearizeAsGain=off  AntiWindupMode=clamping  Kb=1  POutMin=[]  POutMax=[]  IOutMin=[]  IOutMax=[]  DOutMin=[]  DOutMax=[]  NOutMin=[]  NOutMax=[]  SumOutMin=[]  SumOutMax=[]  SaturationOutMin=[]  SaturationOutMax=[]  PParamMin=[]  PParamMax=[]  IParamMin=[]  IParamMax=[]  DParamMin=[]  DParamMax=[]  NParamMin=[]  NParamMax=[]  KbParamMin=[]  KbParamMax=[]  KtParamMin=[]  KtParamMax=[]  KbOutMin=[]  KbOutMax=[]  KtOutMin=[]  KtOutMax=[]  IntegratorOutMin=[]  IntegratorOutMax=[]  FilterOutMin=[]  FilterOutMax=[]  SumI1OutMin=[]  SumI1OutMax=[]  SumI2OutMin=[]  SumI2OutMax=[]  SumI3OutMin=[]  SumI3OutMax=[]  SumI4OutMin=[]  SumI4OutMax=[]  SumDOutMin=[]  SumDOutMax=[]  DifferentiatorOutMin=[]  DifferentiatorOutMax=[]  FilterDiffOutCoefMin=[]  FilterDiffOutCoefMax=[]  ReciprocalOutMin=[]  ReciprocalOutMax=[]  SumDenOutMin=[]  SumDenOutMax=[]  SumNumOutMin=[]  SumNumOutMax=[]  DivideOutMin=[]  DivideOutMax=[]  IntegratorContinuousStateAttributes=''  IntegratorStateMustResolveToSignalObject=off  IntegratorRTWStateStorageClass=Auto  FilterContinuousStateAttributes=''  FilterStateMustResolveToSignalObject=off  FilterRTWStateStorageClass=Auto  ParallelPVariant=InternalParameters  IdealPVariant=Disabled  IVariant=InternalParameters  DVariant=Disabled  IntegratorVariant=Discrete  SatVariant=Enabled  AWVariant=DiscClampingParallel  PCopyVariant=Disabled  TRVariant=Disabled  FdbkBlocksVariant=Forward  IdealPFdbkVariant=Disabled  SatFdbkVariant=Disabled  DerivativeFilterVariant=Disabled  NVariant=Disabled  NCopyVariant=Disabled_SignalSpec  FilterICVariant=Disabled  IntegratorICVariant=InternalICs  ExternalResetVariant=Disabled  TRSumVariant=Passthrough  SumFdbkVariant=Disabled  SumVariant=Sum_PI
  Sum : Sum  Inputs=|+-
  Sum1 : Sum  Inputs=|-+
  Idq_ref : Outport  VectorParamsAs1DForOutWhenUnconnected=off
  wires:
  Demux1/2 -> Sum1/2
  Demux1/1 -> Sum/2
  m/1 -> Demux1/1
  PQref/1 -> Demux/1
  Demux/1 -> Sum/1  "Pref"
  Demux/2 -> Sum1/1  "Qref"
  Reactive Controller/1 -> Mux/2
  Active Controller/1 -> Mux/1
  Mux/1 -> Idq_ref/1
  Sum/1 -> Active Controller/1
  Sum1/1 -> Reactive Controller/1

== system microgridLibrary/Grid-Connected Battery (Multi-mode EMT Model)/Inverter Control/Compute Errors ==
  Vpoc : Inport
  Bus Creator : BusCreator  Inputs=2
  Bus Selector : BusSelector  OutputSignals=Vgrid,Vpoc
  Fourier (Grid) : powerlib_meascontrol/Measurements/Fourier  Freq=Fnom  n=1  InInit=[0, 0]  Ts=Ts_Control
      settings: SourceProductName=Simscape Electrical
  Fourier (Microgrid) : powerlib_meascontrol/Measurements/Fourier  Freq=Fnom  n=1  InInit=[0, 0]  Ts=Ts_Control
      settings: SourceProductName=Simscape Electrical
  Sum1 : Sum  Inputs=|+-
  Sum2 : Sum  Inputs=|+-
  Errors : Outport  VectorParamsAs1DForOutWhenUnconnected=off
  wires:
  Bus Selector/1 -> Fourier (Grid)/1  "<Vgrid>"
  Fourier (Microgrid)/1 -> Sum2/2
  Fourier (Grid)/1 -> Sum2/1
  Vpoc/1 -> Bus Selector/1
  Fourier (Microgrid)/2 -> Sum1/2
  Bus Selector/2 -> Fourier (Microgrid)/1  "<Vpoc>"
  Fourier (Grid)/2 -> Sum1/1
  Bus Creator/1 -> Errors/1
  Sum2/1 -> Bus Creator/1  "MagErr"
  Sum1/1 -> Bus Creator/2  "PhaseErr"

== system microgridLibrary/Grid-Connected Battery (Multi-mode EMT Model)/Inverter Control/Current Control ==
  wt : Inport
  VdVq_meas : Inport  Port=2  PortDimensions=2
  IdIq_meas : Inport  Port=3  PortDimensions=2
  IdIq_ref : Inport  Port=4  PortDimensions=2
  Action Port : ActionPort  InitializeStates=reset
  Current Regulator : Subsystem
  Uabc_ref Generation max (m) = 1 : Subsystem
  Uabc : Outport  VectorParamsAs1DForOutWhenUnconnected=off
  wires:
  wt/1 -> Uabc_ref Generation max (m) = 1/1(wt)
  Current Regulator/1(VdVq_conv) -> Uabc_ref Generation max (m) = 1/2(VdVq_conv)
  VdVq_meas/1 -> Current Regulator/1(VdVq_meas)
  IdIq_meas/1 -> Current Regulator/2(IdIq_meas)
  IdIq_ref/1 -> Current Regulator/3(IdIq_ref)
  Uabc_ref Generation max (m) = 1/1(Uabc_ref) -> Uabc/1

== system microgridLibrary/Grid-Connected Battery (Multi-mode EMT Model)/Inverter Control/PLL & Measurements ==
  note: PLL & Measurements
      | ===================
  Vabc_prim : Inport
  Iabc_prim : Inport  Port=2
  PLL (3ph) : powerlib_meascontrol/PLL/PLL (3ph)  Fmin=45  Par_Init="[-0.57  Fnom]"  ParK=[180, 3200, 1]  TcD=Ts_Control  MaxRateChangeFreq=12  FilterCutOffFreq=25  Ts=Ts_Control  AGC=on
      settings: SourceProductName=Simscape Electrical
  Selector1 : Selector  InputPortWidth=3  IndexOptions=Index vector (dialog)  Indices=[1 2]  OutputSizes=1
  Selector2 : Selector  InputPortWidth=3  IndexOptions=Index vector (dialog)  Indices=[1 2]  OutputSizes=1
  V->pu : Gain  Gain=1/(Vnom_prim*sqrt(2)/sqrt(3))  SaturateOnIntegerOverflow=on  OutDataTypeStr=Inherit: Same as input  ParamDataTypeStr=Inherit: Same as input
  V->pu1 : Gain  Gain=Vnom_prim*sqrt(3)/Pnom/sqrt(2)  SaturateOnIntegerOverflow=on  OutDataTypeStr=Inherit: Same as input  ParamDataTypeStr=Inherit: Same as input
  abc to dq0 : powerlib_meascontrol/Transformations/abc to dq0  Alignment=90 degrees behind phase A axis
      settings: SourceProductName=Simscape Electrical
  abc to dq1 : powerlib_meascontrol/Transformations/abc to dq0  Alignment=90 degrees behind phase A axis
      settings: SourceProductName=Simscape Electrical
  wt : Outport  VectorParamsAs1DForOutWhenUnconnected=off
  VdVq_prim : Outport  Port=2  VectorParamsAs1DForOutWhenUnconnected=off
  IdIq_prim : Outport  Port=3  VectorParamsAs1DForOutWhenUnconnected=off
  tag scope: PLL_Freq=scoped
  wires:
  PLL (3ph)/2 -> abc to dq0/2, abc to dq1/2, wt/1
  Selector1/1 -> IdIq_prim/1
  Selector2/1 -> VdVq_prim/1
  abc to dq0/1 -> Selector2/1
  Iabc_prim/1 -> V->pu1/1
  Vabc_prim/1 -> V->pu/1
  abc to dq1/1 -> Selector1/1
  V->pu/1 -> abc to dq0/1, PLL (3ph)/1
  V->pu1/1 -> abc to dq1/1
  PLL (3ph)/1 -> [PLL_Freq]
